simulink model "magLev_live"  (R2025b)
settings: Solver=ode45  StartTime=0.0  StopTime=10.0  MaxStep=1e-3  RelTol=1e-3
InitFcn:
  | %% Sampling Time of Discrete Control
  | dT = 1e-3; % Sampling Time
  | 
  | %% Parameter of model:
  | param.m = 0.1; % mass
  | param.lambda = 0.1; % linear coefficient
  | param.g = 9.81; % gravity acceleration
  | param.s0 = 0.01; % nomial air gap
libraries: simulink x1, slpidlib x1
settings Model: Creator=pikronthaler  LastModifiedBy=Felix

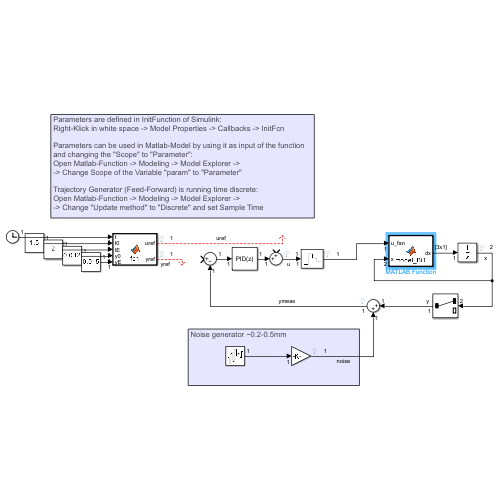
[thumbnail: Simulink's stored preview of the top-level diagram]
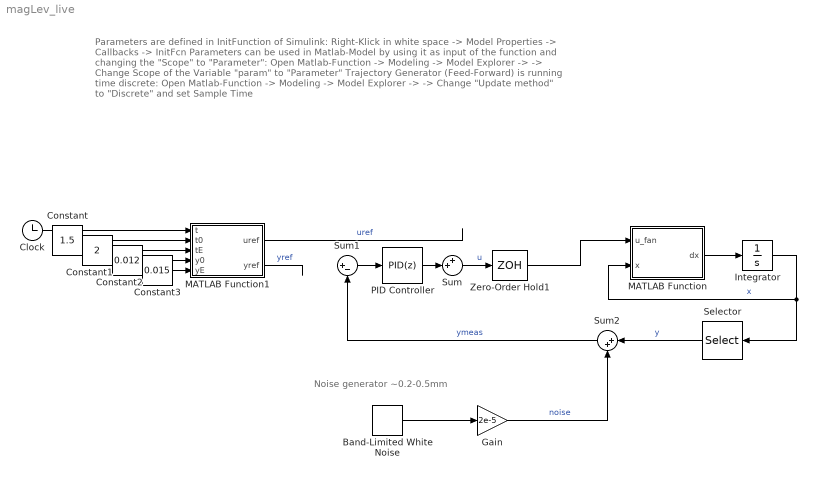
== system magLev_live ==
  note: Parameters are defined in InitFunction of Simulink:
      | Right-Klick in white space -> Model Properties -> Callbacks -> InitFcn
      |
      | Parameters can be used in Matlab-Model by using it as input of the function
      | and changing the "Scope" to "Parameter":
      | Open Matlab-Function -> Modeling -> Model Explorer ->
      | -> Change Scope of the Variable "param" to "Parameter"
      |
      | Trajectory Generator (Feed-Forward) is running time discrete:
      | Open Matlab-Function -> Modeling -> Model Explorer ->
      | -> Change "Update method" to "Discrete" and set Sample Time
  note: Noise generator ~0.2-0.5mm
  Band-Limited White Noise : simulink/Sources/Band-Limited White Noise  Cov=[0.1]  Ts=dT  seed=[23341]
  Clock : Clock
  Constant : Constant  Value=1.5
  Constant1 : Constant  Value=2
  Constant2 : Constant  Value=0.012
  Constant3 : Constant  Value=0.015
  Gain : Gain  Gain=2e-5
  Integrator : Integrator  InitialCondition=[0.012;0]
  MATLAB Function : MATLAB Function  TreatAsAtomicUnit=on
  MATLAB Function1 : MATLAB Function  TreatAsAtomicUnit=on
  PID Controller : slpidlib/PID Controller  Controller=PID  Form=Parallel  TimeDomain=Discrete-time  UseExternalTs=off  SampleTime=dT  IntegratorMethod=Forward Euler  FilterMethod=Forward Euler  ControllerParametersSource=internal  P=0.5  I=0.1  UseKiTs=off  D=0.1  UseExternalDerivativeSource=off  N=100  UseFilter=on  TunerSelectOption=Transfer Function Based (PID Tuner App)  InitialConditionSource=internal  InitialConditionForIntegrator=0  InitialConditionForFilter=0  DifferentiatorICPrevScaledInput=0  ExternalReset=none  TrackingMode=off  Kt=1  LimitOutput=off  SatLimitsSource=internal  UpperSaturationLimit=inf  LowerSaturationLimit=-inf  LinearizeAsGain=on  AntiWindupMode=none  Kb=1  LimitIntegrator=off  UpperIntegratorSaturationLimit=inf  LowerIntegratorSaturationLimit=-inf  POutMin=[]  POutMax=[]  IOutMin=[]  IOutMax=[]  DOutMin=[]  DOutMax=[]  NOutMin=[]  NOutMax=[]  SumOutMin=[]  SumOutMax=[]  SaturationOutMin=[]  SaturationOutMax=[]  PParamMin=[]  PParamMax=[]  IParamMin=[]  IParamMax=[]  DParamMin=[]  DParamMax=[]  NParamMin=[]  NParamMax=[]  KbParamMin=[]  KbParamMax=[]  KtParamMin=[]  KtParamMax=[]  KbOutMin=[]  KbOutMax=[]  KtOutMin=[]  KtOutMax=[]  IntegratorOutMin=[]  IntegratorOutMax=[]  FilterOutMin=[]  FilterOutMax=[]  SumI1OutMin=[]  SumI1OutMax=[]  SumI2OutMin=[]  SumI2OutMax=[]  SumI3OutMin=[]  SumI3OutMax=[]  SumI4OutMin=[]  SumI4OutMax=[]  SumDOutMin=[]  SumDOutMax=[]  DifferentiatorOutMin=[]  DifferentiatorOutMax=[]  FilterDiffOutCoefMin=[]  FilterDiffOutCoefMax=[]  ReciprocalOutMin=[]  ReciprocalOutMax=[]  SumDenOutMin=[]  SumDenOutMax=[]  SumNumOutMin=[]  SumNumOutMax=[]  DivideOutMin=[]  DivideOutMax=[]  UdiffTsProdOutMin=[]  UdiffTsProdOutMax=[]  NTsProdOutMin=[]  NTsProdOutMax=[]  UintegralTsProdOutMin=[]  UintegralTsProdOutMax=[]  UngainTsProdOutMin=[]  UngainTsProdOutMax=[]  ClampingZeroOutDataTypeStr=Inherit: Inherit via back propagation  ClampingZeroOutMin=[]  ClampingZeroOutMax=[]  FilterDenConstantOutDataTypeStr=Inherit: Inherit via back propagation  FilterDenConstantOutMin=[]  FilterDenConstantOutMax=[]  PCopyOutDataTypeStr=Inherit: Inherit via back propagation  PCopyOutMin=[]  PCopyOutMax=[]  NCopyOutDataTypeStr=Inherit: Inherit via back propagation  NCopyOutMin=[]  NCopyOutMax=[]  IntegratorContinuousStateAttributes=''  IntegratorStateMustResolveToSignalObject=off  IntegratorRTWStateStorageClass=Auto  FilterContinuousStateAttributes=''  FilterStateMustResolveToSignalObject=off  FilterRTWStateStorageClass=Auto  ParallelPVariant=InternalParameters  IdealPVariant=Disabled  IVariant=InternalParameters  DVariant=InternalParameters  IntegratorVariant=Discrete  SatVariant=Disabled  AWVariant=Passthrough  PCopyVariant=Disabled  TRVariant=Disabled  FdbkBlocksVariant=Forward  IdealPFdbkVariant=Disabled  SatFdbkVariant=Disabled  DerivativeFilterVariant=ForwardEulerFilter  NVariant=InternalParameters  NCopyVariant=Disabled  FilterICVariant=InternalICsFilter  IntegratorICVariant=InternalICs  ExternalResetVariant=Disabled  TRSumVariant=Passthrough  SumFdbkVariant=Disabled  SumVariant=Sum_PID  TsampFilterVariant=InternalTs  TsampNgainVariant=Passthrough  TsampIntegralVariant=Disabled_SignalSpec  ExternalSaturationOutDataTypeStr=Inherit: Same as second input  DerivativeSourceVariant=ErrorSignal  PreIntVariant=InternalPreInt
  Selector : Selector  InputPortWidth=2  IndexOptions=Index vector (dialog)  Indices=1  OutputSizes=1
  Sum : Sum  Inputs=++|
  Sum1 : Sum  Inputs=|+-
  Sum2 : Sum  Inputs=|++
  Zero-Order Hold1 : ZeroOrderHold  SampleTime=dT
  wires:
  MATLAB Function/1(dx) -> Integrator/1
  Integrator/1 -> Selector/1, MATLAB Function/2(x)  "x"
  PID Controller/1 -> Sum/2
  Sum/1 -> Zero-Order Hold1/1  "u"
  MATLAB Function1/1(uref) -> ?  "uref"
  Sum2/1 -> Sum1/2  "ymeas"
  Sum1/1 -> PID Controller/1
  MATLAB Function1/2(yref) -> ?  "yref"
  Clock/1 -> MATLAB Function1/1(t)
  Constant/1 -> MATLAB Function1/2(t0)
  Constant1/1 -> MATLAB Function1/3(tE)
  Constant2/1 -> MATLAB Function1/4(y0)
  Constant3/1 -> MATLAB Function1/5(yE)
  Selector/1 -> Sum2/1  "y"
  Band-Limited White Noise/1 -> Gain/1
  Gain/1 -> Sum2/2  "noise"
  Zero-Order Hold1/1 -> MATLAB Function/1(u_fan)

== matlab function magLev_live/MATLAB Function1 ==
  settings: updateMethod=DISCRETE  sampleTime=dT
  data: uref output; t input; yref output; t0 input; tE input; y0 input; yE input; param parameter
function [uref,yref] = fcn(t,t0,tE,y0,yE,param)

y = y0;
ydd = 0;

if t>tE
    y = yE;
elseif t>t0
    T = tE-t0;
    tau = (t-t0)/T;
    y = y0+(yE-y0)*(6*tau^5-15*tau^4+10*tau^3);
    yd = (yE-y0)*(30*tau^4-60*tau^3+30*tau^2)*1/T;
    ydd = (yE-y0)*(120*tau^3-180*tau^2+60*tau)*1/T^2;
end

yref = y;
uref = sqrt(param.m*(ydd+param.g)/param.lambda)*(y-param.s0);

== matlab function magLev_live/MATLAB Function ==
  data: u_fan input; x input; dx output
function dx = model_BiT(u_fan, x)
% Define constants as persistent or global variables if running
% outside of a script environment, or simply define them inside
% the function as they are constants.

    alpha1 = 0.0071;
    alpha2 = 0.2237;
    alpha3 = 9.8100;
    u0 = -1.1812;
    tau_w = 1.7217;
    k_w = 286.7462;
    
    % --- Explicitly initialize dx as a 3x1 column vector ---
    % Simulink needs to know the size of this output.
    dx = zeros(3,1); 
    
    % --- State Extraction ---
    x2 = x(2);          % x(2) = dz/dt
    x3 = x(3);          % x(3) = omega (fan speed)
    
    % --- Calculation of State Derivatives ---
    
    % 1. Height derivative (dx1/dt = dz/dt)
    dx(1) = x2; 

    % 2. Velocity derivative (dx2/dt = d^2z/dt^2) - Ball Dynamics
    dx(2) = (alpha1 * x3 - alpha2 * x2)^2 - alpha3;
    
    u_t = (u_fan/100)*5;

    % 3. Fan speed derivative (dx3/dt = d(omega)/dt) - Fan Dynamics
    dx(3) = (1 / tau_w) * (k_w * (u_t - u0) - x3);
    
end
